simulink model "DDCU_wxt_v02_forA_OpenLoop"  (R2014a)
settings: Solver=FixedStepDiscrete  StartTime=0.0  StopTime=16  FixedStep=0.05  RelTol=1e-3
InitFcn:
  | Veh_Par_wxt
values from neighbouring files (symbols this model uses):
  ag_thr = 0.4*g    (= 3.924)    [Veh_Par_wxt.m]
  B = 2.25    [Veh_Par_wxt.m]
  bra_pre_em = 12    [Veh_Par_wxt.m]
  bra_pre_gz2 = 12/3    (= 4)    [Veh_Par_wxt.m]
  bra_pre_gz34 = 12/3    (= 4)    [Veh_Par_wxt.m]
  bra_pre_yd = 12/2    (= 6)    [Veh_Par_wxt.m]
  brakepre_dem_data = [0 1 2 3 4 5 6 7 8 9 10 11 12]    [Veh_Par_wxt.m]
  brakeTrq_dem_data = [0 218.198 436.396 654.594 872.792 1090.99 1309.188 1527.386 1745.584 1963.782 2181.98 2400.178 2618.376]    [Veh_Par_wxt.m]
  bratrq_max = 4*2618.376    (= 10473.504)    [Veh_Par_wxt.m]
  eff_tran = 0.75    [Veh_Par_wxt.m]
  G = Mass*g    (= 36297)    [Veh_Par_wxt.m]
  kd1 = 1    [Veh_Par_wxt.m]
  kd2 = 1    [Veh_Par_wxt.m]
  kd3 = 1    [Veh_Par_wxt.m]
  ki1 = 1    [Veh_Par_wxt.m]
  ki2 = 1    [Veh_Par_wxt.m]
  ki3 = 1    [Veh_Par_wxt.m]
  kp1 = 1    [Veh_Par_wxt.m]
  kp2 = 1    [Veh_Par_wxt.m]
  kp3 = 1    [Veh_Par_wxt.m]
  L = 3.12    [Veh_Par_wxt.m]
  premax = 12    [Veh_Par_wxt.m]
  Radius = 0.20    (= 0.2)    [Veh_Par_wxt.m]
  s_opt_yi_add = 0.05    [Veh_Par_wxt.m]
  s_opt_zhuan_add = 0.05    [Veh_Par_wxt.m]
  spd_map_mot = [0 100 200 300 360 400 500 600 700 800 900]*tras_ratio    [Veh_Par_wxt.m]
  spdmax = 900*tras_ratio    (= 5580)    [Veh_Par_wxt.m]
  speed_thr_park = 5/3.6/Radius*30/pi    (= 66.3145596216)    [Veh_Par_wxt.m]
  tras_ratio = 6.2    [Veh_Par_wxt.m]
  trq_map_mot = [1200 1200 1200 1200 1200 1080 864 720 617 540 480]/tras_ratio    [Veh_Par_wxt.m]
  trqmax = 80    [Veh_Par_wxt.m]
  v_thr1_b = 5    [Veh_Par_wxt.m]
  v_thr2_b = 20    [Veh_Par_wxt.m]
  v_thr_park = 5    [Veh_Par_wxt.m]
undefined symbols (not defined in the file or in its folder): DiscIntNeverNeededParam, sigbuilder_block
libraries: simulink x169, ec5744lib x9
(part 2 of 13)

== system DDCU_wxt_v02_forA_OpenLoop/OutputSignalProcess/VCU_ESC ==
  VVMS_BrkSts_flg_in : Inport
  VVMS_ParkSts_flg_in : Inport  Port=2
  VVMS_BrkPSetLe_MPa_in : Inport  Port=3
  VVMS_BrkPSetRi_MPa_in : Inport  Port=4
  Conv{1..8} (8 alike) : DataTypeConversion
  VCU_ESC_DLC : Constant  Value=8  OutDataTypeStr=uint8
  VCU_ESC_DLC_Out : Terminator
  VCU_ESC_ID : Constant  Value=2364992240  OutDataTypeStr=single
  VCU_ESC_ID_Out : Terminator
  VCU_ESC_mux : Mux  Inputs=8
  VVMS_BrkPSetLe_MPa : Subsystem
  VVMS_BrkPSetRi_MPa : Subsystem
  VVMS_BrkSts_flg : Subsystem
  VVMS_ParkSts_flg : Subsystem
  or{1..8} (8 alike) : simulink/Logic and Bit Operations/Bitwise Operator  logicop=OR  UseBitMask=off  NumInputPorts=4  BitMask=bin2dec('11011001')  BitMaskRealWorld=Stored Integer
  output : Outport
  wires:
  VCU_ESC_mux/1 -> output/1
  VVMS_BrkSts_flg/1(output1) -> or1/1
  VVMS_BrkSts_flg/2(output2) -> or2/1
  VVMS_BrkSts_flg/3(output3) -> or3/1
  VVMS_BrkSts_flg/4(output4) -> or4/1
  VVMS_BrkSts_flg/5(output5) -> or5/1
  VVMS_BrkSts_flg/6(output6) -> or6/1
  VVMS_BrkSts_flg/7(output7) -> or7/1
  VVMS_BrkSts_flg/8(output8) -> or8/1
  VVMS_ParkSts_flg/1(output1) -> or1/2
  VVMS_ParkSts_flg/2(output2) -> or2/2
  VVMS_ParkSts_flg/3(output3) -> or3/2
  VVMS_ParkSts_flg/4(output4) -> or4/2
  VVMS_ParkSts_flg/5(output5) -> or5/2
  VVMS_ParkSts_flg/6(output6) -> or6/2
  VVMS_ParkSts_flg/7(output7) -> or7/2
  VVMS_ParkSts_flg/8(output8) -> or8/2
  VVMS_BrkPSetRi_MPa/1(output1) -> or1/3
  VVMS_BrkPSetRi_MPa/2(output2) -> or2/3
  VVMS_BrkPSetRi_MPa/3(output3) -> or3/3
  VVMS_BrkPSetRi_MPa/4(output4) -> or4/3
  VVMS_BrkPSetRi_MPa/5(output5) -> or5/3
  VVMS_BrkPSetRi_MPa/6(output6) -> or6/3
  VVMS_BrkPSetRi_MPa/7(output7) -> or7/3
  VVMS_BrkPSetRi_MPa/8(output8) -> or8/3
  VVMS_BrkPSetLe_MPa/1(output1) -> or1/4
  VVMS_BrkPSetLe_MPa/2(output2) -> or2/4
  VVMS_BrkPSetLe_MPa/3(output3) -> or3/4
  VVMS_BrkPSetLe_MPa/4(output4) -> or4/4
  VVMS_BrkPSetLe_MPa/5(output5) -> or5/4
  VVMS_BrkPSetLe_MPa/6(output6) -> or6/4
  VVMS_BrkPSetLe_MPa/7(output7) -> or7/4
  VVMS_BrkPSetLe_MPa/8(output8) -> or8/4
  or1/1 -> Conv1/1
  Conv1/1 -> VCU_ESC_mux/1
  or2/1 -> Conv2/1
  Conv2/1 -> VCU_ESC_mux/2
  or3/1 -> Conv3/1
  Conv3/1 -> VCU_ESC_mux/3
  or4/1 -> Conv4/1
  Conv4/1 -> VCU_ESC_mux/4
  or5/1 -> Conv5/1
  Conv5/1 -> VCU_ESC_mux/5
  or6/1 -> Conv6/1
  Conv6/1 -> VCU_ESC_mux/6
  or7/1 -> Conv7/1
  Conv7/1 -> VCU_ESC_mux/7
  or8/1 -> Conv8/1
  Conv8/1 -> VCU_ESC_mux/8
  VCU_ESC_ID/1 -> VCU_ESC_ID_Out/1
  VCU_ESC_DLC/1 -> VCU_ESC_DLC_Out/1
  VVMS_BrkSts_flg_in/1 -> VVMS_BrkSts_flg/1(VVMS_BrkSts_flg)
  VVMS_ParkSts_flg_in/1 -> VVMS_ParkSts_flg/1(VVMS_ParkSts_flg)
  VVMS_BrkPSetRi_MPa_in/1 -> VVMS_BrkPSetRi_MPa/1(VVMS_BrkPSetRi_MPa)
  VVMS_BrkPSetLe_MPa_in/1 -> VVMS_BrkPSetLe_MPa/1(VVMS_BrkPSetLe_MPa)

== system DDCU_wxt_v02_forA_OpenLoop/OutputSignalProcess/VCU_MCU1 ==
  M1Enable_in : Inport
  M1Mode_in : Inport  Port=2
  M1Drive_in : Inport  Port=3
  M1TorqueSet_in : Inport  Port=4
  M1SpeedLimit_in : Inport  Port=5
  M2Enable_in : Inport  Port=6
  M2Mode_in : Inport  Port=7
  M2Drive_in : Inport  Port=8
  M2TorqueSet_in : Inport  Port=9
  M2SpeedLimit_in : Inport  Port=10
  MCU1HeartBeat_in : Inport  Port=11
  Conv{1..8} (8 alike) : DataTypeConversion
  M1Drive : Subsystem
  M1Enable : Subsystem
  M1Mode : Subsystem
  M1SpeedLimit : Subsystem
  M1TorqueSet : Subsystem
  M2Drive : Subsystem
  M2Enable : Subsystem
  M2Mode : Subsystem
  M2SpeedLimit : Subsystem
  M2TorqueSet : Subsystem
  MCU1HeartBeat : Subsystem
  VCU_MCU1_DLC : Constant  Value=8  OutDataTypeStr=uint8
  VCU_MCU1_DLC_Out : Terminator
  VCU_MCU1_ID : Constant  Value=2348937217  OutDataTypeStr=single
  VCU_MCU1_ID_Out : Terminator
  VCU_MCU1_mux : Mux  Inputs=8
  or{1..8} (8 alike) : simulink/Logic and Bit Operations/Bitwise Operator  logicop=OR  UseBitMask=off  NumInputPorts=11  BitMask=bin2dec('11011001')  BitMaskRealWorld=Stored Integer
  output : Outport
  wires:
  VCU_MCU1_mux/1 -> output/1
  MCU1HeartBeat/1(output1) -> or1/1
  MCU1HeartBeat/2(output2) -> or2/1
  MCU1HeartBeat/3(output3) -> or3/1
  MCU1HeartBeat/4(output4) -> or4/1
  MCU1HeartBeat/5(output5) -> or5/1
  MCU1HeartBeat/6(output6) -> or6/1
  MCU1HeartBeat/7(output7) -> or7/1
  MCU1HeartBeat/8(output8) -> or8/1
  M2TorqueSet/1(output1) -> or1/2
  M2TorqueSet/2(output2) -> or2/2
  M2TorqueSet/3(output3) -> or3/2
  M2TorqueSet/4(output4) -> or4/2
  M2TorqueSet/5(output5) -> or5/2
  M2TorqueSet/6(output6) -> or6/2
  M2TorqueSet/7(output7) -> or7/2
  M2TorqueSet/8(output8) -> or8/2
  M2SpeedLimit/1(output1) -> or1/3
  M2SpeedLimit/2(output2) -> or2/3
  M2SpeedLimit/3(output3) -> or3/3
  M2SpeedLimit/4(output4) -> or4/3
  M2SpeedLimit/5(output5) -> or5/3
  M2SpeedLimit/6(output6) -> or6/3
  M2SpeedLimit/7(output7) -> or7/3
  M2SpeedLimit/8(output8) -> or8/3
  M2Mode/1(output1) -> or1/4
  M2Mode/2(output2) -> or2/4
  M2Mode/3(output3) -> or3/4
  M2Mode/4(output4) -> or4/4
  M2Mode/5(output5) -> or5/4
  M2Mode/6(output6) -> or6/4
  M2Mode/7(output7) -> or7/4
  M2Mode/8(output8) -> or8/4
  M2Enable/1(output1) -> or1/5
  M2Enable/2(output2) -> or2/5
  M2Enable/3(output3) -> or3/5
  M2Enable/4(output4) -> or4/5
  M2Enable/5(output5) -> or5/5
  M2Enable/6(output6) -> or6/5
  M2Enable/7(output7) -> or7/5
  M2Enable/8(output8) -> or8/5
  M2Drive/1(output1) -> or1/6
  M2Drive/2(output2) -> or2/6
  M2Drive/3(output3) -> or3/6
  M2Drive/4(output4) -> or4/6
  M2Drive/5(output5) -> or5/6
  M2Drive/6(output6) -> or6/6
  M2Drive/7(output7) -> or7/6
  M2Drive/8(output8) -> or8/6
  M1TorqueSet/1(output1) -> or1/7
  M1TorqueSet/2(output2) -> or2/7
  M1TorqueSet/3(output3) -> or3/7
  M1TorqueSet/4(output4) -> or4/7
  M1TorqueSet/5(output5) -> or5/7
  M1TorqueSet/6(output6) -> or6/7
  M1TorqueSet/7(output7) -> or7/7
  M1TorqueSet/8(output8) -> or8/7
  M1SpeedLimit/1(output1) -> or1/8
  M1SpeedLimit/2(output2) -> or2/8
  M1SpeedLimit/3(output3) -> or3/8
  M1SpeedLimit/4(output4) -> or4/8
  M1SpeedLimit/5(output5) -> or5/8
  M1SpeedLimit/6(output6) -> or6/8
  M1SpeedLimit/7(output7) -> or7/8
  M1SpeedLimit/8(output8) -> or8/8
  M1Mode/1(output1) -> or1/9
  M1Mode/2(output2) -> or2/9
  M1Mode/3(output3) -> or3/9
  M1Mode/4(output4) -> or4/9
  M1Mode/5(output5) -> or5/9
  M1Mode/6(output6) -> or6/9
  M1Mode/7(output7) -> or7/9
  M1Mode/8(output8) -> or8/9
  M1Enable/1(output1) -> or1/10
  M1Enable/2(output2) -> or2/10
  M1Enable/3(output3) -> or3/10
  M1Enable/4(output4) -> or4/10
  M1Enable/5(output5) -> or5/10
  M1Enable/6(output6) -> or6/10
  M1Enable/7(output7) -> or7/10
  M1Enable/8(output8) -> or8/10
  M1Drive/1(output1) -> or1/11
  M1Drive/2(output2) -> or2/11
  M1Drive/3(output3) -> or3/11
  M1Drive/4(output4) -> or4/11
  M1Drive/5(output5) -> or5/11
  M1Drive/6(output6) -> or6/11
  M1Drive/7(output7) -> or7/11
  M1Drive/8(output8) -> or8/11
  or1/1 -> Conv1/1
  Conv1/1 -> VCU_MCU1_mux/1
  or2/1 -> Conv2/1
  Conv2/1 -> VCU_MCU1_mux/2
  or3/1 -> Conv3/1
  Conv3/1 -> VCU_MCU1_mux/3
  or4/1 -> Conv4/1
  Conv4/1 -> VCU_MCU1_mux/4
  or5/1 -> Conv5/1
  Conv5/1 -> VCU_MCU1_mux/5
  or6/1 -> Conv6/1
  Conv6/1 -> VCU_MCU1_mux/6
  or7/1 -> Conv7/1
  Conv7/1 -> VCU_MCU1_mux/7
  or8/1 -> Conv8/1
  Conv8/1 -> VCU_MCU1_mux/8
  VCU_MCU1_ID/1 -> VCU_MCU1_ID_Out/1
  VCU_MCU1_DLC/1 -> VCU_MCU1_DLC_Out/1
  MCU1HeartBeat_in/1 -> MCU1HeartBeat/1(MCU1HeartBeat)
  M2TorqueSet_in/1 -> M2TorqueSet/1(M2TorqueSet)
  M2SpeedLimit_in/1 -> M2SpeedLimit/1(M2SpeedLimit)
  M2Mode_in/1 -> M2Mode/1(M2Mode)
  M2Enable_in/1 -> M2Enable/1(M2Enable)
  M2Drive_in/1 -> M2Drive/1(M2Drive)
  M1TorqueSet_in/1 -> M1TorqueSet/1(M1TorqueSet)
  M1SpeedLimit_in/1 -> M1SpeedLimit/1(M1SpeedLimit)
  M1Mode_in/1 -> M1Mode/1(M1Mode)
  M1Enable_in/1 -> M1Enable/1(M1Enable)
  M1Drive_in/1 -> M1Drive/1(M1Drive)

== matlab function DDCU_wxt_v02_forA_OpenLoop/MainControl/mode_control/forward/forward/Drive/驱动防滑控制TCS/直行TCS/直行/MATLAB Function ==
  data: s_act_lf input; flag_lf output; s_opt_zhuan input; s_opt_zhuan_add input; flag_lf_pre input
function flag_lf = fcn(s_act_lf,s_opt_zhuan,s_opt_zhuan_add,flag_lf_pre)
%#codegen
if s_act_lf>s_opt_zhuan+s_opt_zhuan_add
    flag_lf=1;
elseif s_act_lf<s_opt_zhuan
    flag_lf = 0;
else
    flag_lf=flag_lf_pre;
end
end

== matlab function DDCU_wxt_v02_forA_OpenLoop/MainControl/mode_control/forward/forward/Drive/驱动防滑控制TCS/直行TCS/直行/MATLAB Function4 ==
  data: trq_dem_lf input; trq_dem_lr input; trq_dem_rf input; trq_dem_rr input; bra_pre_l input; bra_pre_r input; brakepre_dem input; flag_lf input; flag_lr input; trq_out_lf output; flag_rf input; flag_rr input; trq_out_lr output; trq_out_rf output; trq_out_rr output; trq_pid_lf input; trq_pid_lr input; trq_pid_rf input; trq_pid_rr input; brapre_out_l output; brapre_out_r output; mode output
function [trq_out_lf,trq_out_lr,trq_out_rf,trq_out_rr,brapre_out_l,brapre_out_r,mode] = fcn(trq_dem_lf,trq_dem_lr,trq_dem_rf,trq_dem_rr,bra_pre_l,bra_pre_r,brakepre_dem,flag_lf,flag_lr,flag_rf,flag_rr,trq_pid_lf,trq_pid_lr,trq_pid_rf,trq_pid_rr)
%#codegen pid模块在外面做，里面进行十六种情况的判断，先看一下效果，不能再修改。
if flag_lf==0 && flag_lr==0 && flag_rf==0 && flag_rr==0 % 0电机滑转===============================================0电机滑转
    trq_out_lf=trq_dem_lf;
    trq_out_lr=trq_dem_lr;
    trq_out_rf=trq_dem_rf;
    trq_out_rr=trq_dem_rr;
    brapre_out_l=bra_pre_l+brakepre_dem;
    brapre_out_r=bra_pre_r+brakepre_dem;
    mode=1;
elseif flag_lf==1 && flag_lr==0 &&flag_rf==0 && flag_rr==0 %左前轮滑转===================================================1电机滑转
    trq_out_lf=trq_pid_lf;
    trq_out_lr=trq_dem_lr+(trq_dem_lf-trq_out_lf);
    trq_out_rf=trq_dem_rf;
    trq_out_rr=trq_dem_rr;
    brapre_out_l=bra_pre_l+brakepre_dem;
    brapre_out_r=bra_pre_r+brakepre_dem;
    mode=2;
elseif flag_lf==0 && flag_lr==1 &&flag_rf==0 && flag_rr==0 %左后轮滑转
    trq_out_lr=trq_pid_lr;
    trq_out_lf=trq_dem_lf+(trq_dem_lr-trq_out_lr);
    trq_out_rf=trq_dem_rf;
    trq_out_rr=trq_dem_rr;
    brapre_out_l=bra_pre_l+brakepre_dem;
    brapre_out_r=bra_pre_r+brakepre_dem;
    mode=3;
elseif flag_lf==0 && flag_lr==0 &&flag_rf==1 && flag_rr==0 %右前轮滑转
    trq_out_rf=trq_pid_rf;
    trq_out_rr=trq_dem_rr+(trq_dem_rf-trq_out_rf);
    trq_out_lf=trq_dem_lf;
    trq_out_lr=trq_dem_lr;
    brapre_out_l=bra_pre_l+brakepre_dem;
    brapre_out_r=bra_pre_r+brakepre_dem;
    mode=4;
elseif flag_lf==0 && flag_lr==0 &&flag_rf==0 && flag_rr==1 %右后轮滑转
    trq_out_rr=trq_pid_rr;
    trq_out_rf=trq_dem_rf+(trq_dem_rr-trq_out_rr);
    trq_out_lf=trq_dem_lf;
    trq_out_lr=trq_dem_lr;
    brapre_out_l=bra_pre_l+brakepre_dem;
    brapre_out_r=bra_pre_r+brakepre_dem;
    mode=5;
elseif flag_lf==1 && flag_lr==1 &&flag_rf==0 && flag_rr==0 %左侧两轮滑转=====================================================================2电机滑转
    trq_out_lf=trq_pid_lf;
    trq_out_lr=trq_pid_lr;
    trq_out_rf=trq_dem_rf-(trq_dem_lf+trq_dem_lr-trq_out_lf-trq_out_lr)/2;
    trq_out_rr=trq_dem_rr-(trq_dem_lf+trq_dem_lr-trq_out_lf-trq_out_lr)/2;
    brapre_out_l=bra_pre_l+brakepre_dem;
    brapre_out_r=bra_pre_r+brakepre_dem;
    mode=6;
elseif flag_lf==0 && flag_lr==0 &&flag_rf==1 && flag_rr==1 %右侧两轮滑转
    trq_out_rf=trq_pid_rf;
    trq_out_rr=trq_pid_rr;
    trq_out_lf=trq_dem_lf-(trq_dem_rf+trq_dem_rr-trq_out_rf-trq_out_rr)/2;
    trq_out_lr=trq_dem_lr-(trq_dem_rf+trq_dem_rr-trq_out_rf-trq_out_rr)/2;
    brapre_out_l=bra_pre_l+brakepre_dem;
    brapre_out_r=bra_pre_r+brakepre_dem;
    mode=7;
elseif flag_lf==1 && flag_lr==0 &&flag_rf==1 && flag_rr==0 %前轴滑转
    trq_out_lf=trq_pid_lf;
    trq_out_lr=trq_dem_lr+(trq_dem_lf-trq_out_lf);
    trq_out_rf=trq_pid_rf;
    trq_out_rr=trq_dem_rr+(trq_dem_rf-trq_out_rf);
    brapre_out_l=bra_pre_l+brakepre_dem;
    brapre_out_r=bra_pre_r+brakepre_dem;
    mode=8;
elseif flag_lf==0 && flag_lr==1 &&flag_rf==0 && flag_rr==1 %后轴滑转
    trq_out_lr=trq_pid_lr;
    trq_out_lf=trq_dem_lf+(trq_dem_lr-trq_out_lr);
    trq_out_rr=trq_pid_rr;
    trq_out_rf=trq_dem_rf+(trq_dem_rr-trq_out_rr);
    brapre_out_l=bra_pre_l+brakepre_dem;
    brapre_out_r=bra_pre_r+brakepre_dem;
    mode=9;
elseif flag_lf==1 && flag_lr==0 &&flag_rf==0 && flag_rr==1 %左前轮和右后轮滑转
    trq_out_lf=trq_pid_lf;
    trq_out_lr=trq_dem_lr+(trq_dem_lf-trq_out_lf);
    trq_out_rr=trq_pid_rr;
    trq_out_rf=trq_dem_rf+(trq_dem_rr-trq_out_rr);
    brapre_out_l=bra_pre_l+brakepre_dem;
    brapre_out_r=bra_pre_r+brakepre_dem;
    mode=10;
elseif flag_lf==0 && flag_lr==1 &&flag_rf==1 && flag_rr==0 %左后轮和右前轮滑转
    trq_out_lr=trq_pid_lr;
    trq_out_lf=trq_dem_lf+(trq_dem_lr-trq_out_lr);
    trq_out_rf=trq_pid_rf;
    trq_out_rr=trq_dem_rr+(trq_dem_rf-trq_out_rf);
    brapre_out_l=bra_pre_l+brakepre_dem;
    brapre_out_r=bra_pre_r+brakepre_dem;
    mode=11;
elseif flag_lf==1 && flag_lr==1 &&flag_rf==1 && flag_rr==0 %右后不滑转======================================================================3电机滑转
    trq_out_lf=trq_pid_lf;
    trq_out_lr=trq_pid_lr;
    trq_out_rf=trq_pid_rf;
    trq_out_rr=trq_dem_rr+(trq_dem_rf-trq_out_rf)-(trq_dem_lf+trq_dem_lr-trq_out_lf-trq_out_lr);
    brapre_out_l=bra_pre_l+brakepre_dem;
    brapre_out_r=bra_pre_r+brakepre_dem;
    mode=12;
elseif flag_lf==1 && flag_lr==1 &&flag_rf==0 && flag_rr==1 %右前不滑转
    trq_out_lf=trq_pid_lf;
    trq_out_lr=trq_pid_lr;
    trq_out_rr=trq_pid_rr;
    trq_out_rf=trq_dem_rf+(trq_dem_rr-trq_out_rr)-(trq_dem_lf+trq_dem_lr-trq_out_lf-trq_out_lr);
    brapre_out_l=bra_pre_l+brakepre_dem;
    brapre_out_r=bra_pre_r+brakepre_dem;
    mode=13;
elseif flag_lf==1 && flag_lr==0 &&flag_rf==1 && flag_rr==1 %左后不滑转
    trq_out_rf=trq_pid_rf;
    trq_out_rr=trq_pid_rr;
    trq_out_lf=trq_pid_lf;
    trq_out_lr=trq_dem_lr+(trq_dem_lf-trq_out_lf)-(trq_dem_rf+trq_dem_rr-trq_out_rf-trq_out_rr);
    brapre_out_l=bra_pre_l+brakepre_dem;
    brapre_out_r=bra_pre_r+brakepre_dem;
    mode=14;
elseif flag_lf==0 && flag_lr==1 &&flag_rf==1 && flag_rr==1 %左前不滑转
    trq_out_rf=trq_pid_rf;
    trq_out_rr=trq_pid_rr;
    trq_out_lr=trq_pid_lr;
    trq_out_lf=trq_dem_lf+(trq_dem_lr-trq_out_lr)-(trq_dem_rf+trq_dem_rr-trq_out_rf-trq_out_rr);
    brapre_out_l=bra_pre_l+brakepre_dem;
    brapre_out_r=bra_pre_r+brakepre_dem;
    mode=15;
else
    %     flag_lf==1 && flag_lr==1 &&flag_rf==1 && flag_rr==1 %4电机均滑转======================================================================4电机均滑转
    trqcha=(trq_pid_lf+trq_pid_lr)-(trq_pid_rf+trq_pid_rr);
    if trqcha>0
        trq_out_rf=trq_pid_rf;
        trq_out_rr=trq_pid_rr;
        trq_out_lf=trq_pid_lf-(trq_pid_lf/(trq_pid_lf+trq_pid_lr))*trqcha;
        trq_out_lr=trq_pid_lr-(trq_pid_lr/(trq_pid_lf+trq_pid_lr))*trqcha;
    else
        trq_out_lf=trq_pid_lf;
        trq_out_lr=trq_pid_lr;
        trq_out_rf=trq_pid_rf+(trq_pid_rf/(trq_pid_rf+trq_pid_rr))*trqcha;
        trq_out_rr=trq_pid_rr+(trq_pid_rr/(trq_pid_rf+trq_pid_rr))*trqcha;
    end
    brapre_out_l=bra_pre_l+brakepre_dem;
    brapre_out_r=bra_pre_r+brakepre_dem;
    mode=16;
end
trq_out_lf=max(0,trq_out_lf);
trq_out_lr=max(0,trq_out_lr);
trq_out_rf=max(0,trq_out_rf);
trq_out_rr=max(0,trq_out_rr);
brapre_out_l=brapre_out_l;
brapre_out_r=brapre_out_r;
end

== system DDCU_wxt_v02_forA_OpenLoop/OutputSignalProcess/VCU_MCU1_replace ==
  M2SpeedSet_in : Inport
  M1SpeedSet_in : Inport  Port=2
  MCU1HeartBeat_in : Inport  Port=3
  M2SpeedLimit_in : Inport  Port=4
  M2Mode_in : Inport  Port=5
  M2Enable_in : Inport  Port=6
  M2Drive_in : Inport  Port=7
  M1SpeedLimit_in : Inport  Port=8
  M1Mode_in : Inport  Port=9
  M1Enable_in : Inport  Port=10
  M1Drive_in : Inport  Port=11
  Conv{1..8} (8 alike) : DataTypeConversion
  M1Drive : Subsystem
  M1Enable : Subsystem
  M1Mode : Subsystem
  M1SpeedLimit : Subsystem
  M1SpeedSet : Subsystem
  M2Drive : Subsystem
  M2Enable : Subsystem
  M2Mode : Subsystem
  M2SpeedLimit : Subsystem
  M2SpeedSet : Subsystem
  MCU1HeartBeat : Subsystem
  VCU_MCU1_replace_DLC : Constant  Value=8  OutDataTypeStr=uint8
  VCU_MCU1_replace_DLC_Out : Terminator
  VCU_MCU1_replace_ID : Constant  Value=2348937233  OutDataTypeStr=single
  VCU_MCU1_replace_ID_Out : Terminator
  VCU_MCU1_replace_mux : Mux  Inputs=8
  or{1..8} (8 alike) : simulink/Logic and Bit Operations/Bitwise Operator  logicop=OR  UseBitMask=off  NumInputPorts=11  BitMask=bin2dec('11011001')  BitMaskRealWorld=Stored Integer
  output : Outport
  wires:
  VCU_MCU1_replace_mux/1 -> output/1
  M2SpeedSet/1(output1) -> or1/1
  M2SpeedSet/2(output2) -> or2/1
  M2SpeedSet/3(output3) -> or3/1
  M2SpeedSet/4(output4) -> or4/1
  M2SpeedSet/5(output5) -> or5/1
  M2SpeedSet/6(output6) -> or6/1
  M2SpeedSet/7(output7) -> or7/1
  M2SpeedSet/8(output8) -> or8/1
  M1SpeedSet/1(output1) -> or1/2
  M1SpeedSet/2(output2) -> or2/2
  M1SpeedSet/3(output3) -> or3/2
  M1SpeedSet/4(output4) -> or4/2
  M1SpeedSet/5(output5) -> or5/2
  M1SpeedSet/6(output6) -> or6/2
  M1SpeedSet/7(output7) -> or7/2
  M1SpeedSet/8(output8) -> or8/2
  MCU1HeartBeat/1(output1) -> or1/3
  MCU1HeartBeat/2(output2) -> or2/3
  MCU1HeartBeat/3(output3) -> or3/3
  MCU1HeartBeat/4(output4) -> or4/3
  MCU1HeartBeat/5(output5) -> or5/3
  MCU1HeartBeat/6(output6) -> or6/3
  MCU1HeartBeat/7(output7) -> or7/3
  MCU1HeartBeat/8(output8) -> or8/3
  M2SpeedLimit/1(output1) -> or1/4
  M2SpeedLimit/2(output2) -> or2/4
  M2SpeedLimit/3(output3) -> or3/4
  M2SpeedLimit/4(output4) -> or4/4
  M2SpeedLimit/5(output5) -> or5/4
  M2SpeedLimit/6(output6) -> or6/4
  M2SpeedLimit/7(output7) -> or7/4
  M2SpeedLimit/8(output8) -> or8/4
  M2Mode/1(output1) -> or1/5
  M2Mode/2(output2) -> or2/5
  M2Mode/3(output3) -> or3/5
  M2Mode/4(output4) -> or4/5
  M2Mode/5(output5) -> or5/5
  M2Mode/6(output6) -> or6/5
  M2Mode/7(output7) -> or7/5
  M2Mode/8(output8) -> or8/5
  M2Enable/1(output1) -> or1/6
  M2Enable/2(output2) -> or2/6
  M2Enable/3(output3) -> or3/6
  M2Enable/4(output4) -> or4/6
  M2Enable/5(output5) -> or5/6
  M2Enable/6(output6) -> or6/6
  M2Enable/7(output7) -> or7/6
  M2Enable/8(output8) -> or8/6
  M2Drive/1(output1) -> or1/7
  M2Drive/2(output2) -> or2/7
  M2Drive/3(output3) -> or3/7
  M2Drive/4(output4) -> or4/7
  M2Drive/5(output5) -> or5/7
  M2Drive/6(output6) -> or6/7
  M2Drive/7(output7) -> or7/7
  M2Drive/8(output8) -> or8/7
  M1SpeedLimit/1(output1) -> or1/8
  M1SpeedLimit/2(output2) -> or2/8
  M1SpeedLimit/3(output3) -> or3/8
  M1SpeedLimit/4(output4) -> or4/8
  M1SpeedLimit/5(output5) -> or5/8
  M1SpeedLimit/6(output6) -> or6/8
  M1SpeedLimit/7(output7) -> or7/8
  M1SpeedLimit/8(output8) -> or8/8
  M1Mode/1(output1) -> or1/9
  M1Mode/2(output2) -> or2/9
  M1Mode/3(output3) -> or3/9
  M1Mode/4(output4) -> or4/9
  M1Mode/5(output5) -> or5/9
  M1Mode/6(output6) -> or6/9
  M1Mode/7(output7) -> or7/9
  M1Mode/8(output8) -> or8/9
  M1Enable/1(output1) -> or1/10
  M1Enable/2(output2) -> or2/10
  M1Enable/3(output3) -> or3/10
  M1Enable/4(output4) -> or4/10
  M1Enable/5(output5) -> or5/10
  M1Enable/6(output6) -> or6/10
  M1Enable/7(output7) -> or7/10
  M1Enable/8(output8) -> or8/10
  M1Drive/1(output1) -> or1/11
  M1Drive/2(output2) -> or2/11
  M1Drive/3(output3) -> or3/11
  M1Drive/4(output4) -> or4/11
  M1Drive/5(output5) -> or5/11
  M1Drive/6(output6) -> or6/11
  M1Drive/7(output7) -> or7/11
  M1Drive/8(output8) -> or8/11
  or1/1 -> Conv1/1
  Conv1/1 -> VCU_MCU1_replace_mux/1
  or2/1 -> Conv2/1
  Conv2/1 -> VCU_MCU1_replace_mux/2
  or3/1 -> Conv3/1
  Conv3/1 -> VCU_MCU1_replace_mux/3
  or4/1 -> Conv4/1
  Conv4/1 -> VCU_MCU1_replace_mux/4
  or5/1 -> Conv5/1
  Conv5/1 -> VCU_MCU1_replace_mux/5
  or6/1 -> Conv6/1
  Conv6/1 -> VCU_MCU1_replace_mux/6
  or7/1 -> Conv7/1
  Conv7/1 -> VCU_MCU1_replace_mux/7
  or8/1 -> Conv8/1
  Conv8/1 -> VCU_MCU1_replace_mux/8
  VCU_MCU1_replace_ID/1 -> VCU_MCU1_replace_ID_Out/1
  VCU_MCU1_replace_DLC/1 -> VCU_MCU1_replace_DLC_Out/1
  M2SpeedSet_in/1 -> M2SpeedSet/1(M2SpeedSet)
  M1SpeedSet_in/1 -> M1SpeedSet/1(M1SpeedSet)
  MCU1HeartBeat_in/1 -> MCU1HeartBeat/1(MCU1HeartBeat)
  M2SpeedLimit_in/1 -> M2SpeedLimit/1(M2SpeedLimit)
  M2Mode_in/1 -> M2Mode/1(M2Mode)
  M2Enable_in/1 -> M2Enable/1(M2Enable)
  M2Drive_in/1 -> M2Drive/1(M2Drive)
  M1SpeedLimit_in/1 -> M1SpeedLimit/1(M1SpeedLimit)
  M1Mode_in/1 -> M1Mode/1(M1Mode)
  M1Enable_in/1 -> M1Enable/1(M1Enable)
  M1Drive_in/1 -> M1Drive/1(M1Drive)

== system DDCU_wxt_v02_forA_OpenLoop/OutputSignalProcess/VCU_MCU2 ==
  M3Enable_in : Inport
  M3Mode_in : Inport  Port=2
  M3Drive_in : Inport  Port=3
  M3TorqueSet_in : Inport  Port=4
  M3SpeedLimit_in : Inport  Port=5
  M4Enable_in : Inport  Port=6
  M4Mode_in : Inport  Port=7
  M4Drive_in : Inport  Port=8
  M4TorqueSet_in : Inport  Port=9
  M4SpeedLimit_in : Inport  Port=10
  MCU2HeartBeat_in : Inport  Port=11
  Conv{1..8} (8 alike) : DataTypeConversion
  M3Drive : Subsystem
  M3Enable : Subsystem
  M3Mode : Subsystem
  M3SpeedLimit : Subsystem
  M3TorqueSet : Subsystem
  M4Drive : Subsystem
  M4Enable : Subsystem
  M4Mode : Subsystem
  M4SpeedLimit : Subsystem
  M4TorqueSet : Subsystem
  MCU2HeartBeat : Subsystem
  VCU_MCU2_DLC : Constant  Value=8  OutDataTypeStr=uint8
  VCU_MCU2_DLC_Out : Terminator
  VCU_MCU2_ID : Constant  Value=2348937218  OutDataTypeStr=single
  VCU_MCU2_ID_Out : Terminator
  VCU_MCU2_mux : Mux  Inputs=8
  or{1..8} (8 alike) : simulink/Logic and Bit Operations/Bitwise Operator  logicop=OR  UseBitMask=off  NumInputPorts=11  BitMask=bin2dec('11011001')  BitMaskRealWorld=Stored Integer
  output : Outport
  wires:
  VCU_MCU2_mux/1 -> output/1
  MCU2HeartBeat/1(output1) -> or1/1
  MCU2HeartBeat/2(output2) -> or2/1
  MCU2HeartBeat/3(output3) -> or3/1
  MCU2HeartBeat/4(output4) -> or4/1
  MCU2HeartBeat/5(output5) -> or5/1
  MCU2HeartBeat/6(output6) -> or6/1
  MCU2HeartBeat/7(output7) -> or7/1
  MCU2HeartBeat/8(output8) -> or8/1
  M4TorqueSet/1(output1) -> or1/2
  M4TorqueSet/2(output2) -> or2/2
  M4TorqueSet/3(output3) -> or3/2
  M4TorqueSet/4(output4) -> or4/2
  M4TorqueSet/5(output5) -> or5/2
  M4TorqueSet/6(output6) -> or6/2
  M4TorqueSet/7(output7) -> or7/2
  M4TorqueSet/8(output8) -> or8/2
  M4SpeedLimit/1(output1) -> or1/3
  M4SpeedLimit/2(output2) -> or2/3
  M4SpeedLimit/3(output3) -> or3/3
  M4SpeedLimit/4(output4) -> or4/3
  M4SpeedLimit/5(output5) -> or5/3
  M4SpeedLimit/6(output6) -> or6/3
  M4SpeedLimit/7(output7) -> or7/3
  M4SpeedLimit/8(output8) -> or8/3
  M4Mode/1(output1) -> or1/4
  M4Mode/2(output2) -> or2/4
  M4Mode/3(output3) -> or3/4
  M4Mode/4(output4) -> or4/4
  M4Mode/5(output5) -> or5/4
  M4Mode/6(output6) -> or6/4
  M4Mode/7(output7) -> or7/4
  M4Mode/8(output8) -> or8/4
  M4Enable/1(output1) -> or1/5
  M4Enable/2(output2) -> or2/5
  M4Enable/3(output3) -> or3/5
  M4Enable/4(output4) -> or4/5
  M4Enable/5(output5) -> or5/5
  M4Enable/6(output6) -> or6/5
  M4Enable/7(output7) -> or7/5
  M4Enable/8(output8) -> or8/5
  M4Drive/1(output1) -> or1/6
  M4Drive/2(output2) -> or2/6
  M4Drive/3(output3) -> or3/6
  M4Drive/4(output4) -> or4/6
  M4Drive/5(output5) -> or5/6
  M4Drive/6(output6) -> or6/6
  M4Drive/7(output7) -> or7/6
  M4Drive/8(output8) -> or8/6
  M3TorqueSet/1(output1) -> or1/7
  M3TorqueSet/2(output2) -> or2/7
  M3TorqueSet/3(output3) -> or3/7
  M3TorqueSet/4(output4) -> or4/7
  M3TorqueSet/5(output5) -> or5/7
  M3TorqueSet/6(output6) -> or6/7
  M3TorqueSet/7(output7) -> or7/7
  M3TorqueSet/8(output8) -> or8/7
  M3SpeedLimit/1(output1) -> or1/8
  M3SpeedLimit/2(output2) -> or2/8
  M3SpeedLimit/3(output3) -> or3/8
  M3SpeedLimit/4(output4) -> or4/8
  M3SpeedLimit/5(output5) -> or5/8
  M3SpeedLimit/6(output6) -> or6/8
  M3SpeedLimit/7(output7) -> or7/8
  M3SpeedLimit/8(output8) -> or8/8
  M3Mode/1(output1) -> or1/9
  M3Mode/2(output2) -> or2/9
  M3Mode/3(output3) -> or3/9
  M3Mode/4(output4) -> or4/9
  M3Mode/5(output5) -> or5/9
  M3Mode/6(output6) -> or6/9
  M3Mode/7(output7) -> or7/9
  M3Mode/8(output8) -> or8/9
  M3Enable/1(output1) -> or1/10
  M3Enable/2(output2) -> or2/10
  M3Enable/3(output3) -> or3/10
  M3Enable/4(output4) -> or4/10
  M3Enable/5(output5) -> or5/10
  M3Enable/6(output6) -> or6/10
  M3Enable/7(output7) -> or7/10
  M3Enable/8(output8) -> or8/10
  M3Drive/1(output1) -> or1/11
  M3Drive/2(output2) -> or2/11
  M3Drive/3(output3) -> or3/11
  M3Drive/4(output4) -> or4/11
  M3Drive/5(output5) -> or5/11
  M3Drive/6(output6) -> or6/11
  M3Drive/7(output7) -> or7/11
  M3Drive/8(output8) -> or8/11
  or1/1 -> Conv1/1
  Conv1/1 -> VCU_MCU2_mux/1
  or2/1 -> Conv2/1
  Conv2/1 -> VCU_MCU2_mux/2
  or3/1 -> Conv3/1
  Conv3/1 -> VCU_MCU2_mux/3
  or4/1 -> Conv4/1
  Conv4/1 -> VCU_MCU2_mux/4
  or5/1 -> Conv5/1
  Conv5/1 -> VCU_MCU2_mux/5
  or6/1 -> Conv6/1
  Conv6/1 -> VCU_MCU2_mux/6
  or7/1 -> Conv7/1
  Conv7/1 -> VCU_MCU2_mux/7
  or8/1 -> Conv8/1
  Conv8/1 -> VCU_MCU2_mux/8
  VCU_MCU2_ID/1 -> VCU_MCU2_ID_Out/1
  VCU_MCU2_DLC/1 -> VCU_MCU2_DLC_Out/1
  MCU2HeartBeat_in/1 -> MCU2HeartBeat/1(MCU2HeartBeat)
  M4TorqueSet_in/1 -> M4TorqueSet/1(M4TorqueSet)
  M4SpeedLimit_in/1 -> M4SpeedLimit/1(M4SpeedLimit)
  M4Mode_in/1 -> M4Mode/1(M4Mode)
  M4Enable_in/1 -> M4Enable/1(M4Enable)
  M4Drive_in/1 -> M4Drive/1(M4Drive)
  M3TorqueSet_in/1 -> M3TorqueSet/1(M3TorqueSet)
  M3SpeedLimit_in/1 -> M3SpeedLimit/1(M3SpeedLimit)
  M3Mode_in/1 -> M3Mode/1(M3Mode)
  M3Enable_in/1 -> M3Enable/1(M3Enable)
  M3Drive_in/1 -> M3Drive/1(M3Drive)

== system DDCU_wxt_v02_forA_OpenLoop/OutputSignalProcess/VCU_MCU2_replace ==
  M4SpeedSet_in : Inport
  M3SpeedSet_in : Inport  Port=2
  MCU2HeartBeat_in : Inport  Port=3
  M4SpeedLimit_in : Inport  Port=4
  M4Mode_in : Inport  Port=5
  M4Enable_in : Inport  Port=6
  M4Drive_in : Inport  Port=7
  M3SpeedLimit_in : Inport  Port=8
  M3Mode_in : Inport  Port=9
  M3Enable_in : Inport  Port=10
  M3Drive_in : Inport  Port=11
  Conv{1..8} (8 alike) : DataTypeConversion
  M3Drive : Subsystem
  M3Enable : Subsystem
  M3Mode : Subsystem
  M3SpeedLimit : Subsystem
  M3SpeedSet : Subsystem
  M4Drive : Subsystem
  M4Enable : Subsystem
  M4Mode : Subsystem
  M4SpeedLimit : Subsystem
  M4SpeedSet : Subsystem
  MCU2HeartBeat : Subsystem
  VCU_MCU2_replace_DLC : Constant  Value=8  OutDataTypeStr=uint8
  VCU_MCU2_replace_DLC_Out : Terminator
  VCU_MCU2_replace_ID : Constant  Value=2348937234  OutDataTypeStr=single
  VCU_MCU2_replace_ID_Out : Terminator
  VCU_MCU2_replace_mux : Mux  Inputs=8
  or{1..8} (8 alike) : simulink/Logic and Bit Operations/Bitwise Operator  logicop=OR  UseBitMask=off  NumInputPorts=11  BitMask=bin2dec('11011001')  BitMaskRealWorld=Stored Integer
  output : Outport
  wires:
  VCU_MCU2_replace_mux/1 -> output/1
  M4SpeedSet/1(output1) -> or1/1
  M4SpeedSet/2(output2) -> or2/1
  M4SpeedSet/3(output3) -> or3/1
  M4SpeedSet/4(output4) -> or4/1
  M4SpeedSet/5(output5) -> or5/1
  M4SpeedSet/6(output6) -> or6/1
  M4SpeedSet/7(output7) -> or7/1
  M4SpeedSet/8(output8) -> or8/1
  M3SpeedSet/1(output1) -> or1/2
  M3SpeedSet/2(output2) -> or2/2
  M3SpeedSet/3(output3) -> or3/2
  M3SpeedSet/4(output4) -> or4/2
  M3SpeedSet/5(output5) -> or5/2
  M3SpeedSet/6(output6) -> or6/2
  M3SpeedSet/7(output7) -> or7/2
  M3SpeedSet/8(output8) -> or8/2
  MCU2HeartBeat/1(output1) -> or1/3
  MCU2HeartBeat/2(output2) -> or2/3
  MCU2HeartBeat/3(output3) -> or3/3
  MCU2HeartBeat/4(output4) -> or4/3
  MCU2HeartBeat/5(output5) -> or5/3
  MCU2HeartBeat/6(output6) -> or6/3
  MCU2HeartBeat/7(output7) -> or7/3
  MCU2HeartBeat/8(output8) -> or8/3
  M4SpeedLimit/1(output1) -> or1/4
  M4SpeedLimit/2(output2) -> or2/4
  M4SpeedLimit/3(output3) -> or3/4
  M4SpeedLimit/4(output4) -> or4/4
  M4SpeedLimit/5(output5) -> or5/4
  M4SpeedLimit/6(output6) -> or6/4
  M4SpeedLimit/7(output7) -> or7/4
  M4SpeedLimit/8(output8) -> or8/4
  M4Mode/1(output1) -> or1/5
  M4Mode/2(output2) -> or2/5
  M4Mode/3(output3) -> or3/5
  M4Mode/4(output4) -> or4/5
  M4Mode/5(output5) -> or5/5
  M4Mode/6(output6) -> or6/5
  M4Mode/7(output7) -> or7/5
  M4Mode/8(output8) -> or8/5
  M4Enable/1(output1) -> or1/6
  M4Enable/2(output2) -> or2/6
  M4Enable/3(output3) -> or3/6
  M4Enable/4(output4) -> or4/6
  M4Enable/5(output5) -> or5/6
  M4Enable/6(output6) -> or6/6
  M4Enable/7(output7) -> or7/6
  M4Enable/8(output8) -> or8/6
  M4Drive/1(output1) -> or1/7
  M4Drive/2(output2) -> or2/7
  M4Drive/3(output3) -> or3/7
  M4Drive/4(output4) -> or4/7
  M4Drive/5(output5) -> or5/7
  M4Drive/6(output6) -> or6/7
  M4Drive/7(output7) -> or7/7
  M4Drive/8(output8) -> or8/7
  M3SpeedLimit/1(output1) -> or1/8
  M3SpeedLimit/2(output2) -> or2/8
  M3SpeedLimit/3(output3) -> or3/8
  M3SpeedLimit/4(output4) -> or4/8
  M3SpeedLimit/5(output5) -> or5/8
  M3SpeedLimit/6(output6) -> or6/8
  M3SpeedLimit/7(output7) -> or7/8
  M3SpeedLimit/8(output8) -> or8/8
  M3Mode/1(output1) -> or1/9
  M3Mode/2(output2) -> or2/9
  M3Mode/3(output3) -> or3/9
  M3Mode/4(output4) -> or4/9
  M3Mode/5(output5) -> or5/9
  M3Mode/6(output6) -> or6/9
  M3Mode/7(output7) -> or7/9
  M3Mode/8(output8) -> or8/9
  M3Enable/1(output1) -> or1/10
  M3Enable/2(output2) -> or2/10
  M3Enable/3(output3) -> or3/10
  M3Enable/4(output4) -> or4/10
  M3Enable/5(output5) -> or5/10
  M3Enable/6(output6) -> or6/10
  M3Enable/7(output7) -> or7/10
  M3Enable/8(output8) -> or8/10
  M3Drive/1(output1) -> or1/11
  M3Drive/2(output2) -> or2/11
  M3Drive/3(output3) -> or3/11
  M3Drive/4(output4) -> or4/11
  M3Drive/5(output5) -> or5/11
  M3Drive/6(output6) -> or6/11
  M3Drive/7(output7) -> or7/11
  M3Drive/8(output8) -> or8/11
  or1/1 -> Conv1/1
  Conv1/1 -> VCU_MCU2_replace_mux/1
  or2/1 -> Conv2/1
  Conv2/1 -> VCU_MCU2_replace_mux/2
  or3/1 -> Conv3/1
  Conv3/1 -> VCU_MCU2_replace_mux/3
  or4/1 -> Conv4/1
  Conv4/1 -> VCU_MCU2_replace_mux/4
  or5/1 -> Conv5/1
  Conv5/1 -> VCU_MCU2_replace_mux/5
  or6/1 -> Conv6/1
  Conv6/1 -> VCU_MCU2_replace_mux/6
  or7/1 -> Conv7/1
  Conv7/1 -> VCU_MCU2_replace_mux/7
  or8/1 -> Conv8/1
  Conv8/1 -> VCU_MCU2_replace_mux/8
  VCU_MCU2_replace_ID/1 -> VCU_MCU2_replace_ID_Out/1
  VCU_MCU2_replace_DLC/1 -> VCU_MCU2_replace_DLC_Out/1
  M4SpeedSet_in/1 -> M4SpeedSet/1(M4SpeedSet)
  M3SpeedSet_in/1 -> M3SpeedSet/1(M3SpeedSet)
  MCU2HeartBeat_in/1 -> MCU2HeartBeat/1(MCU2HeartBeat)
  M4SpeedLimit_in/1 -> M4SpeedLimit/1(M4SpeedLimit)
  M4Mode_in/1 -> M4Mode/1(M4Mode)
  M4Enable_in/1 -> M4Enable/1(M4Enable)
  M4Drive_in/1 -> M4Drive/1(M4Drive)
  M3SpeedLimit_in/1 -> M3SpeedLimit/1(M3SpeedLimit)
  M3Mode_in/1 -> M3Mode/1(M3Mode)
  M3Enable_in/1 -> M3Enable/1(M3Enable)
  M3Drive_in/1 -> M3Drive/1(M3Drive)

== system DDCU_wxt_v02_forA_OpenLoop/OutputSignalProcess/VCU_Park ==
  ParkEnable_in : Inport
  Conv{1..8} (8 alike) : DataTypeConversion
  ParkEnable : Subsystem
  VCU_Park_DLC : Constant  Value=8  OutDataTypeStr=uint8
  VCU_Park_DLC_Out : Terminator
  VCU_Park_ID : Constant  Value=2281988666  OutDataTypeStr=single
  VCU_Park_ID_Out : Terminator
  VCU_Park_mux : Mux  Inputs=8
  or{1..8} (8 alike) : simulink/Logic and Bit Operations/Bitwise Operator  logicop=OR  UseBitMask=off  BitMask=bin2dec('11011001')  BitMaskRealWorld=Stored Integer
  output : Outport
  wires:
  VCU_Park_mux/1 -> output/1
  ParkEnable/1(output1) -> or1/1
  ParkEnable/2(output2) -> or2/1
  ParkEnable/3(output3) -> or3/1
  ParkEnable/4(output4) -> or4/1
  ParkEnable/5(output5) -> or5/1
  ParkEnable/6(output6) -> or6/1
  ParkEnable/7(output7) -> or7/1
  ParkEnable/8(output8) -> or8/1
  or1/1 -> Conv1/1
  Conv1/1 -> VCU_Park_mux/1
  or2/1 -> Conv2/1
  Conv2/1 -> VCU_Park_mux/2
  or3/1 -> Conv3/1
  Conv3/1 -> VCU_Park_mux/3
  or4/1 -> Conv4/1
  Conv4/1 -> VCU_Park_mux/4
  or5/1 -> Conv5/1
  Conv5/1 -> VCU_Park_mux/5
  or6/1 -> Conv6/1
  Conv6/1 -> VCU_Park_mux/6
  or7/1 -> Conv7/1
  Conv7/1 -> VCU_Park_mux/7
  or8/1 -> Conv8/1
  Conv8/1 -> VCU_Park_mux/8
  VCU_Park_ID/1 -> VCU_Park_ID_Out/1
  VCU_Park_DLC/1 -> VCU_Park_DLC_Out/1
  ParkEnable_in/1 -> ParkEnable/1(ParkEnable)

== system DDCU_wxt_v02_forA_OpenLoop/Data_Input/HCU1_VCU/HCU1_VCU ==
  input : Inport
  Enable : EnablePort
  Demux : Demux  Outputs=8
  acc_Ad : Sum
  acc_Convert : DataTypeConversion  OutDataTypeStr=uint32
  acc_F : Gain
  acc_L : simulink/Logic and Bit Operations/Bitwise Operator  logicop=AND  UseBitMask=on  BitMask=65535  BitMaskRealWorld=Stored Integer
  acc_O : Constant  Value=0  OutDataTypeStr=single
  acc_S : ArithShift
  acc_Sub : Subsystem
  acc_sat : Saturate  UpperLimit=65535  LowerLimit=0
  acccv : DataTypeConversion
  accinput2_Ad : Sum
  accinput2_C : Constant  Value=256
  accinput2_P : Product
  break_Ad : Sum
  break_Convert : DataTypeConversion  OutDataTypeStr=uint32
  break_F : Gain
  break_L : simulink/Logic and Bit Operations/Bitwise Operator  logicop=AND  UseBitMask=on  BitMask=255  BitMaskRealWorld=Stored Integer
  break_O : Constant  Value=0  OutDataTypeStr=single
  break_S : ArithShift
  break_Sub : Subsystem
  break_sat : Saturate  UpperLimit=255  LowerLimit=0
  breakcv : DataTypeConversion
  pwr_limit_Ad : Sum
  pwr_limit_Convert : DataTypeConversion  OutDataTypeStr=uint32
  pwr_limit_F : Gain
  pwr_limit_L : simulink/Logic and Bit Operations/Bitwise Operator  logicop=AND  UseBitMask=on  BitMask=255  BitMaskRealWorld=Stored Integer
  pwr_limit_O : Constant  Value=0  OutDataTypeStr=single
  pwr_limit_S : ArithShift
  pwr_limit_Sub : Subsystem
  pwr_limit_sat : Saturate  UpperLimit=255  LowerLimit=0
  pwr_limitcv : DataTypeConversion
  real_velocity_Ad : Sum
  real_velocity_Convert : DataTypeConversion  OutDataTypeStr=uint32
  real_velocity_F : Gain
  real_velocity_L : simulink/Logic and Bit Operations/Bitwise Operator  logicop=AND  UseBitMask=on  BitMask=255  BitMaskRealWorld=Stored Integer
  real_velocity_O : Constant  Value=0  OutDataTypeStr=single
  real_velocity_S : ArithShift
  real_velocity_Sub : Subsystem
  real_velocity_sat : Saturate  UpperLimit=255  LowerLimit=0
  real_velocitycv : DataTypeConversion
  turn_Ad : Sum
  turn_Convert : DataTypeConversion  OutDataTypeStr=uint32
  turn_F : Gain
  turn_L : simulink/Logic and Bit Operations/Bitwise Operator  logicop=AND  UseBitMask=on  BitMask=65535  BitMaskRealWorld=Stored Integer
  turn_O : Constant  Value=0  OutDataTypeStr=single
  turn_S : ArithShift
  turn_Sub : Subsystem
  turn_sat : Saturate  UpperLimit=65535  LowerLimit=0
  turncv : DataTypeConversion
  turninput4_Ad : Sum
  turninput4_C : Constant  Value=256
  turninput4_P : Product
  turn_Out : Outport
  real_velocity_Out : Outport  Port=2
  pwr_limit_Out : Outport  Port=3
  break_Out : Outport  Port=4
  acc_Out : Outport  Port=5
  wires:
  turn_F/1 -> turn_Ad/1
  turn_O/1 -> turn_Ad/2
  turn_Ad/1 -> turn_sat/1
  turn_sat/1 -> turn_Out/1
  Demux/4 -> turninput4_P/1
  turninput4_C/1 -> turninput4_P/2
  turninput4_P/1 -> turninput4_Ad/1
  Demux/3 -> turninput4_Ad/2
  turninput4_Ad/1 -> turn_Sub/1(In1)
  turn_Sub/1(Out1) -> turn_Convert/1
  turn_Convert/1 -> turn_L/1
  turn_L/1 -> turn_S/1
  turn_S/1 -> turncv/1
  turncv/1 -> turn_F/1
  real_velocity_F/1 -> real_velocity_Ad/1
  real_velocity_O/1 -> real_velocity_Ad/2
  real_velocity_Ad/1 -> real_velocity_sat/1
  real_velocity_sat/1 -> real_velocity_Out/1
  Demux/5 -> real_velocity_Sub/1(In1)
  real_velocity_Sub/1(Out1) -> real_velocity_Convert/1
  real_velocity_Convert/1 -> real_velocity_L/1
  real_velocity_L/1 -> real_velocity_S/1
  real_velocity_S/1 -> real_velocitycv/1
  real_velocitycv/1 -> real_velocity_F/1
  pwr_limit_F/1 -> pwr_limit_Ad/1
  pwr_limit_O/1 -> pwr_limit_Ad/2
  pwr_limit_Ad/1 -> pwr_limit_sat/1
  pwr_limit_sat/1 -> pwr_limit_Out/1
  Demux/6 -> pwr_limit_Sub/1(In1)
  pwr_limit_Sub/1(Out1) -> pwr_limit_Convert/1
  pwr_limit_Convert/1 -> pwr_limit_L/1
  pwr_limit_L/1 -> pwr_limit_S/1
  pwr_limit_S/1 -> pwr_limitcv/1
  pwr_limitcv/1 -> pwr_limit_F/1
  break_F/1 -> break_Ad/1
  break_O/1 -> break_Ad/2
  break_Ad/1 -> break_sat/1
  break_sat/1 -> break_Out/1
  Demux/7 -> break_Sub/1(In1)
  break_Sub/1(Out1) -> break_Convert/1
  break_Convert/1 -> break_L/1
  break_L/1 -> break_S/1
  break_S/1 -> breakcv/1
  breakcv/1 -> break_F/1
  acc_F/1 -> acc_Ad/1
  acc_O/1 -> acc_Ad/2
  acc_Ad/1 -> acc_sat/1
  acc_sat/1 -> acc_Out/1
  Demux/2 -> accinput2_P/1
  accinput2_C/1 -> accinput2_P/2
  accinput2_P/1 -> accinput2_Ad/1
  Demux/1 -> accinput2_Ad/2
  accinput2_Ad/1 -> acc_Sub/1(In1)
  acc_Sub/1(Out1) -> acc_Convert/1
  acc_Convert/1 -> acc_L/1
  acc_L/1 -> acc_S/1
  acc_S/1 -> acccv/1
  acccv/1 -> acc_F/1
  input/1 -> Demux/1

== system DDCU_wxt_v02_forA_OpenLoop/Data_Input/HCU1_VCU1/MUC1_VCU1 ==
  input : Inport
  Enable : EnablePort
  Demux : Demux  Outputs=8
  spd_mot_lf_Ad : Sum
  spd_mot_lf_Convert : DataTypeConversion  OutDataTypeStr=uint32
  spd_mot_lf_F : Gain
  spd_mot_lf_L : simulink/Logic and Bit Operations/Bitwise Operator  logicop=AND  UseBitMask=on  BitMask=65535  BitMaskRealWorld=Stored Integer
  spd_mot_lf_O : Constant  Value=0  OutDataTypeStr=single
  spd_mot_lf_S : ArithShift
  spd_mot_lf_Sub : Subsystem
  spd_mot_lf_sat : Saturate  UpperLimit=65535  LowerLimit=0
  spd_mot_lfcv : DataTypeConversion
  spd_mot_lfinput6_Ad : Sum
  spd_mot_lfinput6_C : Constant  Value=256
  spd_mot_lfinput6_P : Product
  spd_mot_lr_Ad : Sum
  spd_mot_lr_Convert : DataTypeConversion  OutDataTypeStr=uint32
  spd_mot_lr_F : Gain
  spd_mot_lr_L : simulink/Logic and Bit Operations/Bitwise Operator  logicop=AND  UseBitMask=on  BitMask=65535  BitMaskRealWorld=Stored Integer
  spd_mot_lr_O : Constant  Value=0  OutDataTypeStr=single
  spd_mot_lr_S : ArithShift
  spd_mot_lr_Sub : Subsystem
  spd_mot_lr_sat : Saturate  UpperLimit=65535  LowerLimit=0
  spd_mot_lrcv : DataTypeConversion
  spd_mot_lrinput8_Ad : Sum
  spd_mot_lrinput8_C : Constant  Value=256
  spd_mot_lrinput8_P : Product
  spd_mot_rf_Ad : Sum
  spd_mot_rf_Convert : DataTypeConversion  OutDataTypeStr=uint32
  spd_mot_rf_F : Gain
  spd_mot_rf_L : simulink/Logic and Bit Operations/Bitwise Operator  logicop=AND  UseBitMask=on  BitMask=65535  BitMaskRealWorld=Stored Integer
  spd_mot_rf_O : Constant  Value=0  OutDataTypeStr=single
  spd_mot_rf_S : ArithShift
  spd_mot_rf_Sub : Subsystem
  spd_mot_rf_sat : Saturate  UpperLimit=65535  LowerLimit=0
  spd_mot_rfcv : DataTypeConversion
  spd_mot_rfinput2_Ad : Sum
  spd_mot_rfinput2_C : Constant  Value=256
  spd_mot_rfinput2_P : Product
  spd_mot_rr_Ad : Sum
  spd_mot_rr_Convert : DataTypeConversion  OutDataTypeStr=uint32
  spd_mot_rr_F : Gain
  spd_mot_rr_L : simulink/Logic and Bit Operations/Bitwise Operator  logicop=AND  UseBitMask=on  BitMask=65535  BitMaskRealWorld=Stored Integer
  spd_mot_rr_O : Constant  Value=0  OutDataTypeStr=single
  spd_mot_rr_S : ArithShift
  spd_mot_rr_Sub : Subsystem
  spd_mot_rr_sat : Saturate  UpperLimit=65535  LowerLimit=0
  spd_mot_rrcv : DataTypeConversion
  spd_mot_rrinput4_Ad : Sum
  spd_mot_rrinput4_C : Constant  Value=256
  spd_mot_rrinput4_P : Product
  spd_mot_rr_Out : Outport
  spd_mot_rf_Out : Outport  Port=2
  spd_mot_lr_Out : Outport  Port=3
  spd_mot_lf_Out : Outport  Port=4
  wires:
  spd_mot_rr_F/1 -> spd_mot_rr_Ad/1
  spd_mot_rr_O/1 -> spd_mot_rr_Ad/2
  spd_mot_rr_Ad/1 -> spd_mot_rr_sat/1
  spd_mot_rr_sat/1 -> spd_mot_rr_Out/1
  Demux/4 -> spd_mot_rrinput4_P/1
  spd_mot_rrinput4_C/1 -> spd_mot_rrinput4_P/2
  spd_mot_rrinput4_P/1 -> spd_mot_rrinput4_Ad/1
  Demux/3 -> spd_mot_rrinput4_Ad/2
  spd_mot_rrinput4_Ad/1 -> spd_mot_rr_Sub/1(In1)
  spd_mot_rr_Sub/1(Out1) -> spd_mot_rr_Convert/1
  spd_mot_rr_Convert/1 -> spd_mot_rr_L/1
  spd_mot_rr_L/1 -> spd_mot_rr_S/1
  spd_mot_rr_S/1 -> spd_mot_rrcv/1
  spd_mot_rrcv/1 -> spd_mot_rr_F/1
  spd_mot_rf_F/1 -> spd_mot_rf_Ad/1
  spd_mot_rf_O/1 -> spd_mot_rf_Ad/2
  spd_mot_rf_Ad/1 -> spd_mot_rf_sat/1
  spd_mot_rf_sat/1 -> spd_mot_rf_Out/1
  Demux/2 -> spd_mot_rfinput2_P/1
  spd_mot_rfinput2_C/1 -> spd_mot_rfinput2_P/2
  spd_mot_rfinput2_P/1 -> spd_mot_rfinput2_Ad/1
  Demux/1 -> spd_mot_rfinput2_Ad/2
  spd_mot_rfinput2_Ad/1 -> spd_mot_rf_Sub/1(In1)
  spd_mot_rf_Sub/1(Out1) -> spd_mot_rf_Convert/1
  spd_mot_rf_Convert/1 -> spd_mot_rf_L/1
  spd_mot_rf_L/1 -> spd_mot_rf_S/1
  spd_mot_rf_S/1 -> spd_mot_rfcv/1
  spd_mot_rfcv/1 -> spd_mot_rf_F/1
  spd_mot_lr_F/1 -> spd_mot_lr_Ad/1
  spd_mot_lr_O/1 -> spd_mot_lr_Ad/2
  spd_mot_lr_Ad/1 -> spd_mot_lr_sat/1
  spd_mot_lr_sat/1 -> spd_mot_lr_Out/1
  Demux/8 -> spd_mot_lrinput8_P/1
  spd_mot_lrinput8_C/1 -> spd_mot_lrinput8_P/2
  spd_mot_lrinput8_P/1 -> spd_mot_lrinput8_Ad/1
  Demux/7 -> spd_mot_lrinput8_Ad/2
  spd_mot_lrinput8_Ad/1 -> spd_mot_lr_Sub/1(In1)
  spd_mot_lr_Sub/1(Out1) -> spd_mot_lr_Convert/1
  spd_mot_lr_Convert/1 -> spd_mot_lr_L/1
  spd_mot_lr_L/1 -> spd_mot_lr_S/1
  spd_mot_lr_S/1 -> spd_mot_lrcv/1
  spd_mot_lrcv/1 -> spd_mot_lr_F/1
  spd_mot_lf_F/1 -> spd_mot_lf_Ad/1
  spd_mot_lf_O/1 -> spd_mot_lf_Ad/2
  spd_mot_lf_Ad/1 -> spd_mot_lf_sat/1
  spd_mot_lf_sat/1 -> spd_mot_lf_Out/1
  Demux/6 -> spd_mot_lfinput6_P/1
  spd_mot_lfinput6_C/1 -> spd_mot_lfinput6_P/2
  spd_mot_lfinput6_P/1 -> spd_mot_lfinput6_Ad/1
  Demux/5 -> spd_mot_lfinput6_Ad/2
  spd_mot_lfinput6_Ad/1 -> spd_mot_lf_Sub/1(In1)
  spd_mot_lf_Sub/1(Out1) -> spd_mot_lf_Convert/1
  spd_mot_lf_Convert/1 -> spd_mot_lf_L/1
  spd_mot_lf_L/1 -> spd_mot_lf_S/1
  spd_mot_lf_S/1 -> spd_mot_lfcv/1
  spd_mot_lfcv/1 -> spd_mot_lf_F/1
  input/1 -> Demux/1

== system DDCU_wxt_v02_forA_OpenLoop/Data_Input/HCU2_VCU/HCU2_VCU ==
  input : Inport
  Enable : EnablePort
  Demux : Demux  Outputs=8
  daodang_Ad : Sum
  daodang_Convert : DataTypeConversion  OutDataTypeStr=uint32
  daodang_F : Gain
  daodang_L : simulink/Logic and Bit Operations/Bitwise Operator  logicop=AND  UseBitMask=on  BitMask=4  BitMaskRealWorld=Stored Integer
  daodang_O : Constant  Value=0  OutDataTypeStr=single
  daodang_S : ArithShift  BitShiftNumber=2
  daodang_Sub : Subsystem
  daodang_sat : Saturate  UpperLimit=1  LowerLimit=0
  daodangcv : DataTypeConversion
  kongdang_Ad : Sum
  kongdang_Convert : DataTypeConversion  OutDataTypeStr=uint32
  kongdang_F : Gain
  kongdang_L : simulink/Logic and Bit Operations/Bitwise Operator  logicop=AND  UseBitMask=on  BitMask=2  BitMaskRealWorld=Stored Integer
  kongdang_O : Constant  Value=0  OutDataTypeStr=single
  kongdang_S : ArithShift  BitShiftNumber=1
  kongdang_Sub : Subsystem
  kongdang_sat : Saturate  UpperLimit=1  LowerLimit=0
  kongdangcv : DataTypeConversion
  qianjin_Ad : Sum
  qianjin_Convert : DataTypeConversion  OutDataTypeStr=uint32
  qianjin_F : Gain
  qianjin_L : simulink/Logic and Bit Operations/Bitwise Operator  logicop=AND  UseBitMask=on  BitMask=1  BitMaskRealWorld=Stored Integer
  qianjin_O : Constant  Value=0  OutDataTypeStr=single
  qianjin_S : ArithShift
  qianjin_Sub : Subsystem
  qianjin_sat : Saturate  UpperLimit=1  LowerLimit=0
  qianjincv : DataTypeConversion
  zhongxinzhuanxiang_Ad : Sum
  zhongxinzhuanxiang_Convert : DataTypeConversion  OutDataTypeStr=uint32
  zhongxinzhuanxiang_F : Gain
  zhongxinzhuanxiang_L : simulink/Logic and Bit Operations/Bitwise Operator  logicop=AND  UseBitMask=on  BitMask=8  BitMaskRealWorld=Stored Integer
  zhongxinzhuanxiang_O : Constant  Value=0  OutDataTypeStr=single
  zhongxinzhuanxiang_S : ArithShift  BitShiftNumber=3
  zhongxinzhuanxiang_Sub : Subsystem
  zhongxinzhuanxiang_sat : Saturate  UpperLimit=1  LowerLimit=0
  zhongxinzhuanxiangcv : DataTypeConversion
  zhuche_Ad : Sum
  zhuche_Convert : DataTypeConversion  OutDataTypeStr=uint32
  zhuche_F : Gain
  zhuche_L : simulink/Logic and Bit Operations/Bitwise Operator  logicop=AND  UseBitMask=on  BitMask=16  BitMaskRealWorld=Stored Integer
  zhuche_O : Constant  Value=0  OutDataTypeStr=single
  zhuche_S : ArithShift  BitShiftNumber=4
  zhuche_Sub : Subsystem
  zhuche_sat : Saturate  UpperLimit=1  LowerLimit=0
  zhuchecv : DataTypeConversion
  zhuche_Out : Outport
  zhongxinzhuanxiang_Out : Outport  Port=2
  qianjin_Out : Outport  Port=3
  kongdang_Out : Outport  Port=4
  daodang_Out : Outport  Port=5
  wires:
  zhuche_F/1 -> zhuche_Ad/1
  zhuche_O/1 -> zhuche_Ad/2
  zhuche_Ad/1 -> zhuche_sat/1
  zhuche_sat/1 -> zhuche_Out/1
  Demux/1 -> qianjin_Sub/1(In1), daodang_Sub/1(In1), zhongxinzhuanxiang_Sub/1(In1), zhuche_Sub/1(In1), kongdang_Sub/1(In1)
  zhuche_Sub/1(Out1) -> zhuche_Convert/1
  zhuche_Convert/1 -> zhuche_L/1
  zhuche_L/1 -> zhuche_S/1
  zhuche_S/1 -> zhuchecv/1
  zhuchecv/1 -> zhuche_F/1
  zhongxinzhuanxiang_F/1 -> zhongxinzhuanxiang_Ad/1
  zhongxinzhuanxiang_O/1 -> zhongxinzhuanxiang_Ad/2
  zhongxinzhuanxiang_Ad/1 -> zhongxinzhuanxiang_sat/1
  zhongxinzhuanxiang_sat/1 -> zhongxinzhuanxiang_Out/1
  zhongxinzhuanxiang_Sub/1(Out1) -> zhongxinzhuanxiang_Convert/1
  zhongxinzhuanxiang_Convert/1 -> zhongxinzhuanxiang_L/1
  zhongxinzhuanxiang_L/1 -> zhongxinzhuanxiang_S/1
  zhongxinzhuanxiang_S/1 -> zhongxinzhuanxiangcv/1
  zhongxinzhuanxiangcv/1 -> zhongxinzhuanxiang_F/1
  qianjin_F/1 -> qianjin_Ad/1
  qianjin_O/1 -> qianjin_Ad/2
  qianjin_Ad/1 -> qianjin_sat/1
  qianjin_sat/1 -> qianjin_Out/1
  qianjin_Sub/1(Out1) -> qianjin_Convert/1
  qianjin_Convert/1 -> qianjin_L/1
  qianjin_L/1 -> qianjin_S/1
  qianjin_S/1 -> qianjincv/1
  qianjincv/1 -> qianjin_F/1
  kongdang_F/1 -> kongdang_Ad/1
  kongdang_O/1 -> kongdang_Ad/2
  kongdang_Ad/1 -> kongdang_sat/1
  kongdang_sat/1 -> kongdang_Out/1
  kongdang_Sub/1(Out1) -> kongdang_Convert/1
  kongdang_Convert/1 -> kongdang_L/1
  kongdang_L/1 -> kongdang_S/1
  kongdang_S/1 -> kongdangcv/1
  kongdangcv/1 -> kongdang_F/1
  daodang_F/1 -> daodang_Ad/1
  daodang_O/1 -> daodang_Ad/2
  daodang_Ad/1 -> daodang_sat/1
  daodang_sat/1 -> daodang_Out/1
  daodang_Sub/1(Out1) -> daodang_Convert/1
  daodang_Convert/1 -> daodang_L/1
  daodang_L/1 -> daodang_S/1
  daodang_S/1 -> daodangcv/1
  daodangcv/1 -> daodang_F/1
  input/1 -> Demux/1

== system DDCU_wxt_v02_forA_OpenLoop/MainControl/mode_control/Park ==
  Signals : Inport
  Action Port : ActionPort  ActionType=case
  Mux : Mux  Inputs=6
  park : Subsystem
  park_dem : Outport
  wires:
  Signals/1 -> park/1(Signals)
  park/4(mot_rr) -> Mux/4
  park/3(mot_rf) -> Mux/3
  park/5(bra_pre_l) -> Mux/5
  park/2(mot_lr) -> Mux/2
  park/6(bra_pre_r) -> Mux/6
  park/1(mot_lf) -> Mux/1
  Mux/1 -> park_dem/1

== system DDCU_wxt_v02_forA_OpenLoop/MainControl/mode_control/backward ==
  Signals : Inport
  Action Port : ActionPort  ActionType=case
  backward : Subsystem
  backward_dem : Outport
  wires:
  Signals/1 -> backward/1(Signals)
  backward/1(backward_dem) -> backward_dem/1

== system DDCU_wxt_v02_forA_OpenLoop/MainControl/mode_control/center_steer ==
  Signals : Inport
  Action Port : ActionPort  ActionType=case
  Mux : Mux  Inputs=6
  center_steer : Subsystem
  center_steer_dem : Outport
  wires:
  Mux/1 -> center_steer_dem/1
  center_steer/6(bra_pre_r) -> Mux/6
  center_steer/5(bra_pre_l) -> Mux/5
  Signals/1 -> center_steer/1(Signals)
  center_steer/1(mot_lf) -> Mux/1
  center_steer/2(mot_lr) -> Mux/2
  center_steer/4(mot_rr) -> Mux/4
  center_steer/3(mot_rf) -> Mux/3

== system DDCU_wxt_v02_forA_OpenLoop/MainControl/mode_control/emergency_stop ==
  Signals : Inport
  Action Port : ActionPort  ActionType=case
  Mux : Mux  Inputs=6
  emergency_stop : Subsystem
  emergency_stop_dem : Outport
  wires:
  Mux/1 -> emergency_stop_dem/1
  emergency_stop/1(mot_lf) -> Mux/1
  emergency_stop/6(bra_pre_r) -> Mux/6
  emergency_stop/4(mot_rr) -> Mux/4
  emergency_stop/5(bra_pre_l) -> Mux/5
  emergency_stop/3(mot_rf) -> Mux/3
  emergency_stop/2(mot_lr) -> Mux/2
  Signals/1 -> emergency_stop/1(Signals)

== system DDCU_wxt_v02_forA_OpenLoop/MainControl/mode_control/forward ==
  Signals : Inport
  Action Port : ActionPort  ActionType=case
  forward : Subsystem
  forward_dem : Outport
  wires:
  forward/1(forward_dem) -> forward_dem/1
  Signals/1 -> forward/1(Signals)

== system DDCU_wxt_v02_forA_OpenLoop/MainControl/mode_control/neutral ==
  Signals : Inport
  Action Port : ActionPort  ActionType=case
  Mux : Mux  Inputs=6
  neutral : Subsystem
  neutral_dem : Outport
  wires:
  Mux/1 -> neutral_dem/1
  Signals/1 -> neutral/1(Signals)
  neutral/2(mot_lr) -> Mux/2
  neutral/3(mot_rf) -> Mux/3
  neutral/1(mot_lf) -> Mux/1
  neutral/6(bra_pre_r) -> Mux/6
  neutral/5(bra_pre_l) -> Mux/5
  neutral/4(mot_rr) -> Mux/4
